simulink model "Gyro_Outage_Unit_Test"  (R2018b)
settings: Solver=VariableStepAuto  StartTime=0.0  StopTime=5600  FixedStep=fswParams.sample_time_s  RelTol=1e-8  AbsTol=1e-8
undefined symbols (not defined in the file or in its folder): B_eci_unit, Conversion_lib, DiscIntNeverNeededParam, e2sun_eci_unit, ECLIPSE, env_acc_mps2, Environment_lib, fswParams, gyro_body_radps, gyro_meas_valid, mag_body_T, mag_meas_valid, MEKF_Conversion_lib, MEKF_lib, photodiodes_A, q_body, r_eci_km, satelliteDynamics_lib, sc2sun_eci_unit, Sensors_Lib, simParams, solar_panel_power_W, sun_sensor_lib, sunsensor_2body_lib, sunsensor_body_deg, sunsensor_body_rad, sunsensor_valid, Triad, Triad_lib, v_eci_km, w_body_radps
libraries: aerolibutil x11, vrlib x10, sharedutil x8, simulink x5, dspmathops x4, sharedtransform x3, magnetometer_lib x3, gyroscope_lib x2, gravityGrad_Lib x1, atmoDrag_lib x1, magField_lib x1, solarPressure_lib x1
(part 3 of 3)

== system Gyro_Outage_Unit_Test/Sensors_Lib/gyroscope_array/gyroscope_lib ==
  note: check the value of omega against
      | the programmed measurement range
      | of the sensor
  omega_in_radps : Inport
  ARW : Gain  Gain=simParams.sensors.gyro.arw(id_s)
  Cast To Double : DataTypeConversion  OutDataTypeStr=double
  Check Static Range : simulink/Model Verification/Check  Static Range  Description=simParams.sensors.gyro.w_min(id_s) <= u <= simParams.sensors.gyro.w_max(id_s)  max=simParams.sensors.gyro.w_max(id_s)  max_included=on  min=simParams.sensors.gyro.w_min(id_s)  min_included=on  enabled=on  stopWhenAssertionFail=off  export=on  icon=graphic
      settings: SourceProductName=Simulink  SourceProductBaseCode=SL
  Check Static Range1 : simulink/Model Verification/Check  Static Range  Description=simParams.sensors.gyro.w_min(id_s) <= u <= simParams.sensors.gyro.w_max(id_s)  max=simParams.sensors.gyro.w_max(id_s)  max_included=on  min=simParams.sensors.gyro.w_min(id_s)  min_included=on  enabled=on  stopWhenAssertionFail=off  export=on  icon=graphic
      settings: SourceProductName=Simulink  SourceProductBaseCode=SL
  Check Static Range2 : simulink/Model Verification/Check  Static Range  Description=simParams.sensors.gyro.w_min(id_s) <= u <= simParams.sensors.gyro.w_max(id_s)  max=simParams.sensors.gyro.w_max(id_s)  max_included=on  min=simParams.sensors.gyro.w_min(id_s)  min_included=on  enabled=on  stopWhenAssertionFail=off  export=on  icon=graphic
      settings: SourceProductName=Simulink  SourceProductBaseCode=SL
  Demux : Demux  Outputs=3
  Discrete-Time Integrator : DiscreteIntegrator  InitialCondition=simParams.sensors.gyro.bias_init(id_s)  SampleTime=-1  ICPrevOutput=DiscIntNeverNeededParam  ICPrevScaledInput=DiscIntNeverNeededParam
  Logical Operator : Logic  Inputs=3  AllPortsSameDT=off  OutDataTypeStr=boolean
  Quantizer1 : Quantizer  QuantizationInterval=simParams.sensors.gyro.resolution(id_s)
  Quantizer2 : Quantizer  QuantizationInterval=simParams.sensors.gyro.resolution(id_s)
  RRW : Gain  Gain=simParams.sensors.gyro.rrw(id_s)
  Random Number : RandomNumber  Mean=[0 0 0]  Variance=[1 1 1]  Seed=simParams.sensors.gyro.seed_arw(:,id_s)  SampleTime=simParams.sensors.gyro.sample_time_s
  Random Number1 : RandomNumber  Mean=[0 0 0]  Variance=[1 1 1]  Seed=simParams.sensors.gyro.seed_rrw(:,id_s)  SampleTime=simParams.sensors.gyro.sample_time_s
  Rate Transition : RateTransition  InitialCondition=simParams.initialConditions.w0  OutPortSampleTime=simParams.sensors.gyro.sample_time_s
  Rate Transition1 : RateTransition  InitialCondition=simParams.initialConditions.w0
  Rate Transition2 : RateTransition  InitialCondition=simParams.sensors.gyro.bias_init(id_s)
  Rate Transition3 : RateTransition  InitialCondition=1
  Scope : Scope
  Sum : Sum  Inputs=|++
  Sum1 : Sum  Inputs=|++
  omega_radps : Outport
  bias_out : Outport  Port=2
  gyro_valid : Outport  Port=3
  wires:
  Logical Operator/1 -> Cast To Double/1
  Check Static Range2/1 -> Logical Operator/3
  Check Static Range/1 -> Logical Operator/1
  Check Static Range1/1 -> Logical Operator/2
  Demux/1 -> Check Static Range/1
  Demux/2 -> Check Static Range1/1
  Demux/3 -> Check Static Range2/1
  Rate Transition3/1 -> gyro_valid/1
  Rate Transition2/1 -> bias_out/1
  Rate Transition1/1 -> Scope/1, omega_radps/1
  Rate Transition/1 -> Sum/1, Demux/1
  Quantizer2/1 -> Rate Transition1/1
  Sum1/1 -> Quantizer2/1
  Quantizer1/1 -> Sum/2
  Discrete-Time Integrator/1 -> Sum1/2, Rate Transition2/1
  Cast To Double/1 -> Rate Transition3/1
  RRW/1 -> Discrete-Time Integrator/1
  Sum/1 -> Sum1/1
  omega_in_radps/1 -> Rate Transition/1
  ARW/1 -> Quantizer1/1
  Random Number1/1 -> RRW/1
  Random Number/1 -> ARW/1

== system Gyro_Outage_Unit_Test/Sensors_Lib/sun_sensor_lib /deg_err ==
  note: Computes the norm of the 2x1 degree error vector
  angles_meas : Inport
  angles_true : Inport  Port=2
  Dot Product : DotProduct  InputSameDT=on  OutDataTypeStr=Inherit: Inherit via internal rule
  Sqrt : Sqrt  SaturateOnIntegerOverflow=on
  Sum : Sum  Inputs=+-
  deg_err : Outport
  wires:
  Sqrt/1 -> deg_err/1
  Dot Product/1 -> Sqrt/1
  Sum/1 -> Dot Product/1, Dot Product/2
  angles_true/1 -> Sum/2
  angles_meas/1 -> Sum/1

== system Gyro_Outage_Unit_Test/Sensors_Lib/sun_sensor_lib /degree_err ==
  Mux : Mux  Inputs=2
  Random Number2 : RandomNumber  Variance=simParams.sensors.sun_sensor.deg_var  Seed=simParams.sensors.sun_sensor.seed(1)  SampleTime=simParams.sensors.sun_sensor.sample_time_s
  Random Number3 : RandomNumber  Variance=simParams.sensors.sun_sensor.deg_var  Seed=simParams.sensors.sun_sensor.seed(2)  SampleTime=simParams.sensors.sun_sensor.sample_time_s
  "err_deg " : Outport
  wires:
  Mux/1 -> "err_deg "/1
  Random Number3/1 -> Mux/2
  Random Number2/1 -> Mux/1

== system Gyro_Outage_Unit_Test/satelliteDynamics_lib/RigidBodyDynamics/dynamics ==
  note: Euler's equation: J dw/dt = T_{ext} + T_{rw} - w x ( Jw + h_w )
      |
      | RW being momentum exchange devices do NOT create
      | an external torque on the s/c
  external_torque_Nm : Inport
  rw_torque_Nm : Inport  Port=2
  rw_momentum_Nms : Inport  Port=3
  omega_radps : Inport  Port=4
  Add : Sum  Inputs=|++
  Cross Product : vrlib/Utilities/Cross Product
      settings: SourceProductBaseCode=VR
  Invert  3x3 Matrix : aerolibutil/Invert  3x3 Matrix
  Product : Product  Multiplication=Matrix(*)  RndMeth=Zero
  Product1 : Product  Multiplication=Matrix(*)  RndMeth=Zero
  Sum : Sum  Inputs=+-+
  inertia_tensor1 : Constant  Value=simParams.scParams.J
  inertia_tensor2 : Constant  Value=simParams.scParams.J
  omega_dot : Outport
  wires:
  rw_momentum_Nms/1 -> Add/2
  external_torque_Nm/1 -> Sum/1
  omega_radps/1 -> Product/2, Cross Product/1
  inertia_tensor2/1 -> Product/1
  Sum/1 -> Product1/2
  Product1/1 -> omega_dot/1
  Invert  3x3 Matrix/1 -> Product1/1
  inertia_tensor1/1 -> Invert  3x3 Matrix/1
  Cross Product/1 -> Sum/2
  Product/1 -> Add/1
  Add/1 -> Cross Product/2
  rw_torque_Nm/1 -> Sum/3

== system Gyro_Outage_Unit_Test/MEKF_lib1/Measurement Update/Subsystem/Cross_product_matrix2 ==
  sun_body_hat : Inport
  Constant1 : Constant  Value=0
  Constant2 : Constant  Value=0
  Constant3 : Constant  Value=0
  Demux1 : Demux  Outputs=3
  Gain1 : Gain  Gain=-1
  Gain3 : Gain  Gain=-1
  Gain4 : Gain  Gain=-1
  Makes Cross Product Matrix : Reshape  OutputDimensionality=Customize  OutputDimensions=[3,3]
  Vector Concatenate : Concatenate  NumInputs=9
  sun_body_x : Outport
  wires:
  Gain1/1 -> Vector Concatenate/8
  Gain4/1 -> Vector Concatenate/4
  [v2] -> Gain3/1
  Constant1/1 -> Vector Concatenate/1
  [v1] -> Gain1/1
  Gain3/1 -> Vector Concatenate/3
  sun_body_hat/1 -> Demux1/1
  [v3] -> Vector Concatenate/2
  [v2] -> Vector Concatenate/7
  Demux1/2 -> [v2]
  Constant2/1 -> Vector Concatenate/5
  Vector Concatenate/1 -> Makes Cross Product Matrix/1
  Demux1/3 -> [v3]
  [v3] -> Gain4/1
  Constant3/1 -> Vector Concatenate/9
  [v1] -> Vector Concatenate/6
  Demux1/1 -> [v1]
  Makes Cross Product Matrix/1 -> sun_body_x/1

== system Gyro_Outage_Unit_Test/MEKF_lib1/Measurement Update/Subsystem/Cross_product_matrix3 ==
  mag_body_hat : Inport
  Constant1 : Constant  Value=0
  Constant2 : Constant  Value=0
  Constant3 : Constant  Value=0
  Demux1 : Demux  Outputs=3
  Gain1 : Gain  Gain=-1
  Gain3 : Gain  Gain=-1
  Gain4 : Gain  Gain=-1
  Makes Cross Product Matrix : Reshape  OutputDimensionality=Customize  OutputDimensions=[3,3]
  Vector Concatenate : Concatenate  NumInputs=9
  mag_body_x : Outport
  wires:
  mag_body_hat/1 -> Demux1/1
  [v1] -> Vector Concatenate/6
  [v2] -> Vector Concatenate/7
  Gain3/1 -> Vector Concatenate/3
  [v3] -> Gain4/1
  [v3] -> Vector Concatenate/2
  Demux1/1 -> [v1]
  Gain1/1 -> Vector Concatenate/8
  Constant1/1 -> Vector Concatenate/1
  [v1] -> Gain1/1
  Makes Cross Product Matrix/1 -> mag_body_x/1
  Demux1/3 -> [v3]
  Constant2/1 -> Vector Concatenate/5
  Vector Concatenate/1 -> Makes Cross Product Matrix/1
  Demux1/2 -> [v2]
  Gain4/1 -> Vector Concatenate/4
  Constant3/1 -> Vector Concatenate/9
  [v2] -> Gain3/1

== system Gyro_Outage_Unit_Test/MEKF_lib1/Time Propagation (q,P)/Psi/If Action Subsystem ==
  del_t : Inport
  omega_vec : Inport  Port=2
  omega_mag : Inport  Port=3
  Action Port : ActionPort  ActionType=else
  Constant : Constant  Value=0.5
  Divide : Product  Inputs=***
  Divide1 : Product  Inputs=**/
  Sin : Trigonometry
  Psi : Outport
  wires:
  Divide1/1 -> Psi/1  "Psi"
  omega_mag/1 -> Divide1/3, Divide/3
  Constant/1 -> Divide/2
  omega_vec/1 -> Divide1/2
  Divide/1 -> Sin/1
  del_t/1 -> Divide/1
  Sin/1 -> Divide1/1  "sin(om_mag*0.5*del_t)"

== system Gyro_Outage_Unit_Test/MEKF_lib1/Time Propagation (q,P)/Psi/If Action Subsystem1 ==
  Action Port : ActionPort  ActionType=then
  Constant : Constant  Value=0
  Constant1 : Constant  Value=0
  Constant2 : Constant  Value=0
  Mux : Mux  Inputs=3
  Psi_zero : Outport
  wires:
  Constant/1 -> Mux/1
  Constant1/1 -> Mux/2
  Constant2/1 -> Mux/3
  Mux/1 -> Psi_zero/1

== system Gyro_Outage_Unit_Test/MEKF_lib2/Measurement Update/Subsystem/Cross_product_matrix2 ==
  sun_body_hat : Inport
  Constant1 : Constant  Value=0
  Constant2 : Constant  Value=0
  Constant3 : Constant  Value=0
  Demux1 : Demux  Outputs=3
  Gain1 : Gain  Gain=-1
  Gain3 : Gain  Gain=-1
  Gain4 : Gain  Gain=-1
  Makes Cross Product Matrix : Reshape  OutputDimensionality=Customize  OutputDimensions=[3,3]
  Vector Concatenate : Concatenate  NumInputs=9
  sun_body_x : Outport
  wires:
  Makes Cross Product Matrix/1 -> sun_body_x/1
  Demux1/1 -> [v1]
  [v1] -> Vector Concatenate/6
  Constant3/1 -> Vector Concatenate/9
  [v3] -> Gain4/1
  Demux1/3 -> [v3]
  Vector Concatenate/1 -> Makes Cross Product Matrix/1
  Constant2/1 -> Vector Concatenate/5
  Demux1/2 -> [v2]
  [v2] -> Vector Concatenate/7
  [v3] -> Vector Concatenate/2
  sun_body_hat/1 -> Demux1/1
  Gain3/1 -> Vector Concatenate/3
  [v1] -> Gain1/1
  Constant1/1 -> Vector Concatenate/1
  [v2] -> Gain3/1
  Gain4/1 -> Vector Concatenate/4
  Gain1/1 -> Vector Concatenate/8

== system Gyro_Outage_Unit_Test/MEKF_lib2/Measurement Update/Subsystem/Cross_product_matrix3 ==
  mag_body_hat : Inport
  Constant1 : Constant  Value=0
  Constant2 : Constant  Value=0
  Constant3 : Constant  Value=0
  Demux1 : Demux  Outputs=3
  Gain1 : Gain  Gain=-1
  Gain3 : Gain  Gain=-1
  Gain4 : Gain  Gain=-1
  Makes Cross Product Matrix : Reshape  OutputDimensionality=Customize  OutputDimensions=[3,3]
  Vector Concatenate : Concatenate  NumInputs=9
  mag_body_x : Outport
  wires:
  [v2] -> Gain3/1
  Constant3/1 -> Vector Concatenate/9
  Gain4/1 -> Vector Concatenate/4
  Demux1/2 -> [v2]
  Vector Concatenate/1 -> Makes Cross Product Matrix/1
  Constant2/1 -> Vector Concatenate/5
  Demux1/3 -> [v3]
  Makes Cross Product Matrix/1 -> mag_body_x/1
  [v1] -> Gain1/1
  Constant1/1 -> Vector Concatenate/1
  Gain1/1 -> Vector Concatenate/8
  Demux1/1 -> [v1]
  [v3] -> Vector Concatenate/2
  [v3] -> Gain4/1
  Gain3/1 -> Vector Concatenate/3
  [v2] -> Vector Concatenate/7
  [v1] -> Vector Concatenate/6
  mag_body_hat/1 -> Demux1/1

== system Gyro_Outage_Unit_Test/MEKF_lib2/Time Propagation (q,P)/Psi/If Action Subsystem ==
  del_t : Inport
  omega_vec : Inport  Port=2
  omega_mag : Inport  Port=3
  Action Port : ActionPort  ActionType=else
  Constant : Constant  Value=0.5
  Divide : Product  Inputs=***
  Divide1 : Product  Inputs=**/
  Sin : Trigonometry
  Psi : Outport
  wires:
  Sin/1 -> Divide1/1  "sin(om_mag*0.5*del_t)"
  del_t/1 -> Divide/1
  Divide/1 -> Sin/1
  omega_vec/1 -> Divide1/2
  Constant/1 -> Divide/2
  omega_mag/1 -> Divide/3, Divide1/3
  Divide1/1 -> Psi/1  "Psi"

== system Gyro_Outage_Unit_Test/MEKF_lib2/Time Propagation (q,P)/Psi/If Action Subsystem1 ==
  Action Port : ActionPort  ActionType=then
  Constant : Constant  Value=0
  Constant1 : Constant  Value=0
  Constant2 : Constant  Value=0
  Mux : Mux  Inputs=3
  Psi_zero : Outport
  wires:
  Mux/1 -> Psi_zero/1
  Constant2/1 -> Mux/3
  Constant1/1 -> Mux/2
  Constant/1 -> Mux/1

== matlab function Gyro_Outage_Unit_Test/satelliteDynamics_lib/quat_propagation/MATLAB Function ==
  data: w input; Omega output
function Omega = skew_sym(w)
%#codegen

    w_skew = ...
        [0 w(3) -w(2);
        -w(3) 0 w(1);
        w(2) -w(1) 0];

    Omega = ...
        [0 -w';
        w w_skew];

== matlab function Gyro_Outage_Unit_Test/MEKF_lib1/MEKF or Propagation/Angle_between_vectors/MATLAB Function ==
  data: u input; y output
function y = fcn(u)
%#codegen
if abs(u) <=  cosd(2.5)
    y = 1;
else
y = 0;
end

== matlab function Gyro_Outage_Unit_Test/MEKF_lib1/Triad/Angle_between_vectors/MATLAB Function ==
  data: u input; y output
function y = fcn(u)
%#codegen
if abs(u) <=  cosd(2.5)
    y = 1;
else
y = 0;
end

== matlab function Gyro_Outage_Unit_Test/MEKF_lib2/Angle_between_vectors/MATLAB Function ==
  data: u input; y output
function y = fcn(u)
%#codegen
if abs(u) <=  0.9983
    y = 1;
else
y = 0;
end

== matlab function Gyro_Outage_Unit_Test/MEKF_lib2/Measurement Update/MATLAB Function ==
  data: P_sq output; R_sq input; K output; P_sq input; gyro_valid input; H input
function [P_sq,K] = fcnAQR(R_sq,P_sq, gyro_valid,H)
%#codegen
[nr,~] = size(R_sq);
[np,~] = size(P_sq);
A_QR = [R_sq',zeros(nr,np);(P_sq')*H', P_sq'];

[~,R] = qr(A_QR);
        P_sq = R(7:12,7:12)'; %Updated P_sq
        K_bar = R(1:6,7:12)';    
        Innovation_sq = R(1:6,1:6)';
        
        K = K_bar/(Innovation_sq);
        
        if( gyro_valid == 0 )
    K(4:6,:) = zeros(3,6); %this is done so that we do not update bias based
                            % on false gyro readings
        end
end

== matlab function Gyro_Outage_Unit_Test/MEKF_lib2/Measurement Update/P, Kalman Gain ==
  data: R input; Pplus output size=[6,6]; Pminus input; gyro_valid input; H input; K output size=[6,6]
function [Pplus,K] = fcn113(R,Pminus,gyro_valid,H)
K = Pminus*H'/(H*Pminus*H' + R);

if( gyro_valid == 0 )
    K(4:6,:) = zeros(3,6); %this is done so that we do not update bias based
                            % on false gyro readings
end

        KHI = (K*H - eye(6));
        Pplus= KHI*Pminus*KHI' + K*R*K';
end

== matlab function Gyro_Outage_Unit_Test/MEKF_lib2/Time Propagation (q,P)/MATLAB Function ==
  data: P_sq input; Phi_discrete input; P_sq output; Q_sq input
function P_sq  = Cqr(P_sq,Phi_discrete,Q_sq)
%#codegen

A_QR2 = [P_sq'*Phi_discrete';Q_sq'];
         [~,R2] = qr(A_QR2);
          sq_P_kp1 = R2(1:6,1:6)';
          P_sq = sq_P_kp1;
end

== matlab function Gyro_Outage_Unit_Test/MEKF_lib2/Time Propagation (q,P)/MATLAB Function1 ==
  data: Phi input; P_plus1 output; Pk_min input; Q_k input
function P_plus1 = fcn(Phi,Pk_min,Q_k)
%#codegen

P_plus1 = Phi*Pk_min*Phi' + Q_k;

== matlab function Gyro_Outage_Unit_Test/MEKF_lib2/Time Propagation (q,P)/MATLAB Function10 ==
  data: om_mag input; omega_x input; dt input; Phi output
function Phi = Phi_disc(om_mag,omega_x,dt)
%#codegen
% State Transition Matrix
w_n     = om_mag;
w_skew  = omega_x;

if( w_n < 1e-10 )
    Phi = [ eye(3)     -eye(3)*dt;
            zeros(3,3)  eye(3) ];
else
    Phi_11  = eye(3) - w_skew*(sin(w_n*dt)/w_n) + ...
                                        w_skew^2*(1 - cos(w_n*dt))/w_n^2;
    Phi_12  = w_skew*(1 - cos(w_n*dt))/w_n^2 - eye(3)*dt - ...
                                    w_skew^2*(w_n*dt - sin(w_n*dt))/w_n^3;
    Phi_21  = zeros(3,3);    
    Phi_22  = eye(3);    
    Phi     = [ Phi_11 Phi_12;
                Phi_21 Phi_22 ];
end

== matlab function Gyro_Outage_Unit_Test/MEKF_lib1/Measurement Update/QR Factorization ==
  data: P_sq output; R_sq input; K output; P_sq input; gyro_valid input; H input
function [P_sq,K] = A_QR(R_sq,P_sq, gyro_valid,H)
%#codegen
[nr,~] = size(R_sq);
[np,~] = size(P_sq);
A_QR = [R_sq',zeros(nr,np);(P_sq')*H', P_sq'];

[~,R] = qr(A_QR);
        P_sq = R(7:12,7:12)'; %Updated P_sq
        K_bar = R(1:6,7:12)';    
        Innovation_sq = R(1:6,1:6)';
        
        K = K_bar/(Innovation_sq);
        
        if( gyro_valid == 0 )
    K(4:6,:) = zeros(3,6); %this is done so that we do not update bias based
                            % on false gyro readings
        end
end

== matlab function Gyro_Outage_Unit_Test/MEKF_lib1/Time Propagation (q,P)/MATLAB Function10 ==
  data: om_mag input; omega_x input; dt input; Phi output
function Phi = Phi_disc(om_mag,omega_x,dt)
%#codegen
% State Transition Matrix
w_n     = om_mag;
w_skew  = omega_x;

if( w_n < 1e-10 )
    Phi = [ eye(3)     -eye(3)*dt;
            zeros(3,3)  eye(3) ];
else
    Phi_11  = eye(3) - w_skew*(sin(w_n*dt)/w_n) + ...
                                        w_skew^2*(1 - cos(w_n*dt))/w_n^2;
    Phi_12  = w_skew*(1 - cos(w_n*dt))/w_n^2 - eye(3)*dt - ...
                                    w_skew^2*(w_n*dt - sin(w_n*dt))/w_n^3;
    Phi_21  = zeros(3,3);    
    Phi_22  = eye(3);    
    Phi     = [ Phi_11 Phi_12;
                Phi_21 Phi_22 ];
end

== matlab function Gyro_Outage_Unit_Test/MEKF_lib1/Time Propagation (q,P)/MATLAB Function ==
  data: P_sq input; Phi_discrete input; P_sq output; Q_sq input
function P_sq  = Cqr(P_sq,Phi_discrete,Q_sq)
%#codegen

A_QR2 = [P_sq'*Phi_discrete';Q_sq'];
         [~,R2] = qr(A_QR2);
          sq_P_kp1 = R2(1:6,1:6)';
          P_sq = sq_P_kp1;
end
